simulink model "cars_following"  (R2020a)
settings: Solver=VariableStepAuto  StartTime=0.0  StopTime=10.0  RelTol=1e-3
settings Model: Creator=Khojasteh Mirza  LastModifiedBy=Khojasteh Mirza
settings DebuggingCC: UnderSpecifiedDimensionMsg=warning

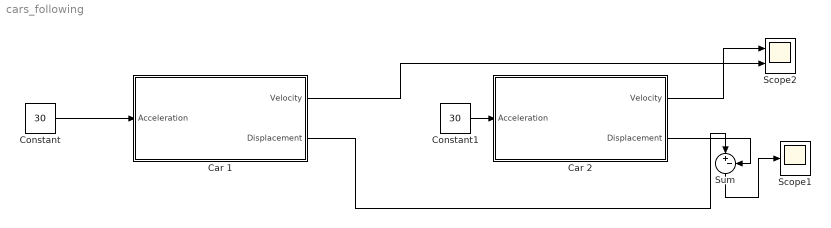
== system cars_following ==
  Car 1 : Subsystem  mask{Pos=100, Vel=10}
      mask prompts: Pos "initial position"; Vel "initial velocity"
      mask TypeOptions Pos: initial displacement/Value
      mask TypeOptions Vel: initial velocity/Value
  Car 2 : Subsystem  mask{Pos=100, Vel=10}
      mask prompts: Pos "initial position"; Vel "initial velocity"
      mask TypeOptions Pos: initial displacement/Value
      mask TypeOptions Vel: initial velocity/Value
  Constant : Constant  Value=30
  Constant1 : Constant  Value=30
  Scope1 : Scope
  Scope2 : Scope  NumInputPorts=2
  Sum : Sum  Inputs=|+-
  wires:
  Constant/1 -> Car 1/1(Acceleration)
  Constant1/1 -> Car 2/1(Acceleration)
  Car 1/1("Velocity ") -> Scope2/2
  Car 2/2(Displacement) -> Sum/2
  Car 1/2(Displacement) -> Sum/1
  Sum/1 -> Scope1/1
  Car 2/1("Velocity ") -> Scope2/1

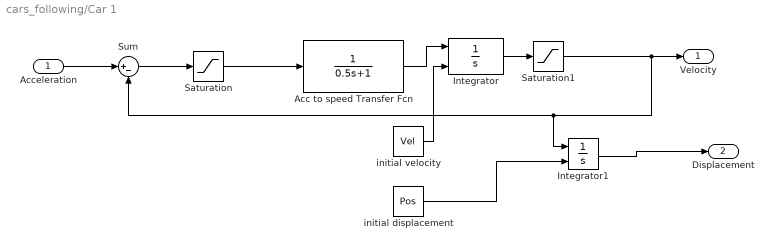
== system cars_following/Car 1 ==
  Acceleration : Inport
  Acc to speed Transfer Fcn : TransferFcn  Denominator=[0.5 1]
  Integrator : Integrator  InitialConditionSource=external
  Integrator1 : Integrator  InitialConditionSource=external
  Saturation : Saturate  UpperLimit=3  LowerLimit=-3
  Saturation1 : Saturate  UpperLimit=inf  LowerLimit=0
  Sum : Sum  Inputs=|+-
  initial displacement : Constant  Value=Pos
  initial velocity : Constant  Value=Vel
  "Velocity " : Outport
  Displacement : Outport  Port=2
  wires:
  Saturation1/1 -> "Velocity "/1, Integrator1/1, Sum/2
  Saturation/1 -> Acc to speed Transfer Fcn/1
  initial velocity/1 -> Integrator/2
  Integrator/1 -> Saturation1/1
  Integrator1/1 -> Displacement/1
  Acc to speed Transfer Fcn/1 -> Integrator/1
  initial displacement/1 -> Integrator1/2
  Sum/1 -> Saturation/1
  Acceleration/1 -> Sum/1

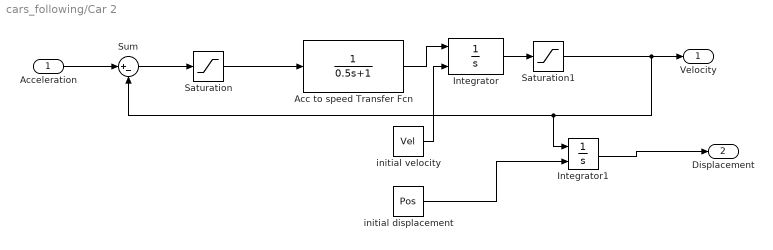
== system cars_following/Car 2 ==
  Acceleration : Inport
  Acc to speed Transfer Fcn : TransferFcn  Denominator=[0.5 1]
  Integrator : Integrator  InitialConditionSource=external
  Integrator1 : Integrator  InitialConditionSource=external
  Saturation : Saturate  UpperLimit=3  LowerLimit=-3
  Saturation1 : Saturate  UpperLimit=inf  LowerLimit=0
  Sum : Sum  Inputs=|+-
  initial displacement : Constant  Value=Pos
  initial velocity : Constant  Value=Vel
  "Velocity " : Outport
  Displacement : Outport  Port=2
  wires:
  Acceleration/1 -> Sum/1
  Sum/1 -> Saturation/1
  initial displacement/1 -> Integrator1/2
  Acc to speed Transfer Fcn/1 -> Integrator/1
  Integrator1/1 -> Displacement/1
  Integrator/1 -> Saturation1/1
  initial velocity/1 -> Integrator/2
  Saturation/1 -> Acc to speed Transfer Fcn/1
  Saturation1/1 -> Sum/2, Integrator1/1, "Velocity "/1
